simulink model "sm_flex_fe_import_beam_test"  (R2016a)
settings: Solver=ode23t  SolverMode=SingleTasking  StartTime=0.0  StopTime=tip_force_duration*2  RelTol=1e-3  AbsTol=1e-3
PreLoadFcn:
  | if(~exist('beamLink','var'))
  | sm_flex_fe_import_params
  | end
PostLoadFcn:
  | sm_flex_fe_import_beam_configure_load(bdroot,'Tip Load');
undefined symbols (not defined in the file): beamLink, gravity_vector, tip_force, tip_force_duration
libraries: nesl_utility x7, sm_lib x4, sm_flex_body_lib x1
CloseFcn:
  | try,close(h1_sm_flex_fe_import_beam),end
  | clear h1_sm_flex_fe_import_beam
  | try,close(h2_sm_flex_fe_import_beam),end
  | clear h2_sm_flex_fe_import_beam
  | try,close(h3_sm_flex_fe_import_beam),end
  | clear h3_sm_flex_fe_import_beam
  | try,close(h4_sm_flex_fe_import_beam),end
  | clear h4_sm_flex_fe_import_beam
  | 
  | 
  | clear simlog_sm_flex_fe_import_beam
  | clear logsout_sm_flex_fe_import_beam
Description:
  | Flexible Beam from Finite Element Data
  | 
  | Copyright 2016-2017 The MathWorks, Inc.
settings Model: Creator=yvanwedd  LastModifiedBy=smiller
settings DataIOCC: MaxDataPoints=25000  SignalLoggingName=logsout_sm_flex_fe_import_beam
settings DebuggingCC: SFUnexpectedBacktrackingDiag=error  SFNoUnconditionalDefaultTransitionDiag=error
settings GRTTargetCC: TargetLangStandard=C99 (ISO)  GeneratePreprocessorConditionals=Use local settings
settings ConfigComp: CovMetricSettings=dwe  CovHtmlReporting=off  CovSaveCumulativeToWorkspaceVar=off  CovSaveSingleToWorkspaceVar=off  CovExternalEMLEnable=on
settings SimscapeCC: SimscapeLogType=all  SimscapeLogSimulationStatistics=on  SimscapeLogName=simlog_sm_flex_fe_import_beam  SimscapeLogDataHistory=25000
settings ExplorerConfigSet: InternalSimMechanicsExplorerSettings="<ExplorerConfiguration><canonicalview>default</canonicalview><AnimationSetting><BasePlaybackSpeed>1.0</BasePlaybackSpeed><PlaybackSpeedFactor>4.0</PlaybackSpeedFactor></AnimationSetting><TilePanel><TileInfo><Tiles Columns=\"1\" Count=\"1\" Rows=\"1\"><Column Left=\"2\" Weight=\"1\"/><Column Left=\"597\"/><Row Top=\"2\" Weight=\"1\"/><Row Top=\"485\"/><Tile Height=\"1\" Width=\"1\" X=\"0\" Y=\"0\"/></Tiles></TileInfo><SceneInfo><SceneViewer><BGColor><R>1</R><G>1</G><B>1</B></BGColor><Camera><DoPerspective>off</DoPerspective><Position><X>1.1286167496242077</X><Y>0.14530787779879978</Y><Z>-0.1353875216555199</Z></Position><Center><X>0.14961601353852311</X><Y>-0.0070840019085978458</Y><Z>1.6591069809918091e-05</Z></Center><Up><X>-0.15237300927665429</X><Y>0.98826658924766431</Y><Z>0.010564782097399028</Z></Up><ViewLimDist>1</ViewLimDist><YLim>0.037474021129310135</YLim><XLim>0.046328642155645021</XLim></Camera></SceneViewer></SceneInfo></TilePanel><MechEditorPanel><Cameras/><GfxPanelCameraMap/><VideoCreator><PlaybackSpeedRatio>1.0</PlaybackSpeedRatio><FrameRate>30</FrameRate><VideoFormat>Motion JPEG AVI</VideoFormat><FrameSize>auto</FrameSize></VideoCreator></MechEditorPanel></ExplorerConfiguration>"

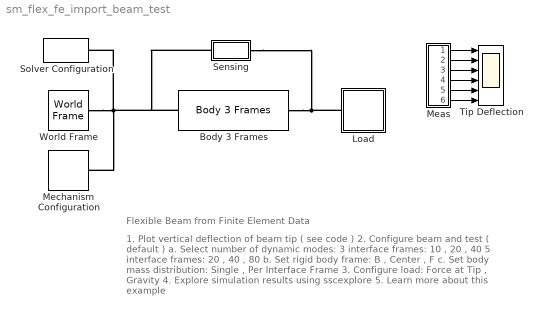
== system sm_flex_fe_import_beam_test ==
  note: Flexible Beam from Finite Element Data
  note: 1. Plot vertical deflection of beam tip ( see code )
      | 2. Configure beam and test ( default )
      | a. Select number of dynamic modes:
      | 3 interface frames: 10 , 20 , 40
      | 5 interface frames: 20 , 40 , 80
      | b. Set rigid body frame: B , Center , F
      | c. Set body mass distribution: Single , Per Interface Frame
      | 3. Configure load: Force at Tip , Gravity
      | 4. Explore simulation results using sscexplore
      | 5. Learn more about this example
  Body 3 Frames : sm_flex_body_lib/FE Import/Bodies/Body 3 Frames  popup_massdistr=Per Interface Frame  mass=beamLink.iner.mass  com=beamLink.iner.com  moi=beamLink.iner.moi  poi=beamLink.iner.poi  splitBodyProps=beamLink.splitBodyProps(2).props  smallInertiaDim=1e-3  smallInertiaMass=1e-6  rigid_body_filename='BeamLink.stl'  rigid_body_color=[0.0 0.4 0.6]  rigid_body_opacity=0  intf_body_color=[0.0 0.4 0.6]  intf_body_opacity=1  intf_graphic_color=[0.0 0.4 0.6]  intf_graphic_opacity=0  rigidBodyFrame=2  T=beamLink.models(5).T  numframes=3  K=beamLink.models(5).K  M=beamLink.models(5).M  ksi=0.05  dofIdxMap=beamLink.models(5).dofIdxMap  tau=1e-6  H=beamLink.models(5).H  sensedFeaDofs_UI=[]  numDynModes=20
      settings: AttributesFormatString=|
      | Mass: %<popup_massdistr>
      | Interface Frames: %<numframes>
      | Rigid Frame: %<rigidBodyFrame>
      | # Dynamic Modes: %<numDynModes>
  Load : Subsystem  mask{t1=0, t2=tip_force_duration, A=tip_force, loadDir=fy, coefs_dl=beamLink.coefs.cdf, coefs=beamLink.coefs.ctl, beam_mass=beamLink.iner.mass, grav_vector=gravity_vector}
      mask prompts: t1 "Start Time (sec)"; t2 "End Time (sec)"; A "Magnitude"; loadDir "Load Direction"; coefs_dl "Distributed Load Coefficients"; coefs "Tip Load Coefficients"; beam_mass "Beam Mass (kg)"; grav_vector "Gravity [x y z] (m/s^2)"
      mask init:
      | blk = [gcb '/External Force and Torque'];
      | mult_x = 0; mult_tx = 0;
      | mult_y = 0; mult_ty = 0;
      | mult_z = 0; mult_tz = 0;
      | 
      | switch loadDir
      |     case 1,
      |         set_param(blk, 'EnableForceX', 'on');
      |         set_param(blk, 'EnableForceY', 'off');
      |         set_param(blk, 'EnableForceZ', 'off');
      |         set_param(blk, 'EnableTorqueX', 'off');
      |         set_param(blk, 'EnableTorqueY', 'off');
      |         set_param(blk, 'EnableTorqueZ', 'off');
      |         mult_x = 1;
      |     case 2,
      |         set_param(blk, 'EnableForceY', 'on');
      |         set_param(blk, 'EnableForceX', 'off');
      |         set_param(blk, 'EnableForceZ', 'off');
      |         set_param(blk, 'EnableTorqueX', 'off');
      |         set_param(blk, 'EnableTorqueY', 'off');
      |         set_param(blk, 'EnableTorqueZ', 'off');
      |         mult_y = 1;
      |     case 3,
      |         set_param(blk, 'EnableForceZ', 'on');
      |         set_param(blk, 'EnableForceX', 'off');
      |         set_param(blk, 'EnableForceY', 'off');
      |         set_param(blk, 'EnableTorqueX', 'off');
      |         set_param(blk, 'EnableTorqueY', 'off');
      |         set_param(blk, 'EnableTorqueZ', 'off');
      |         mult_z = 1;
      |     case 4,
      |         set_param(blk, 'EnableTorqueX', 'on');
      |         set_param(blk, 'EnableForceX', 'off');
      |         set_param(blk, 'EnableForceY', 'off');
      |         set_param(blk, 'EnableForceZ', 'off');
      |         set_param(blk, 'EnableTorqueY', 'off');
      |         set_param(blk, 'EnableTorqueZ', 'off');
      |         mult_tx = 1;
      |     case 5,
      |         set_param(blk, 'EnableTorqueY', 'on');
      |         set_param(blk, 'EnableForceX', 'off');
      |         set_param(blk, 'EnableForceY', 'off');
      |         set_param(blk, 'EnableForceZ', 'off');
      |         set_param(blk, 'EnableTorqueX', 'off');
      |         set_param(blk, 'EnableTorqueZ', 'off');
      |         mult_ty = 1;
      |     case 6,
      |         set_param(blk, 'EnableTorqueZ', 'on');
      |         set_param(blk, 'EnableForceX', 'off');
      |         set_param(blk, 'EnableForceY', 'off');
      |         set_param(blk, 'EnableForceZ', 'off');
      |         set_param(blk, 'EnableTorqueX', 'off');
      |         set_param(blk, 'EnableTorqueY', 'off');
      |         mult_tz = 1;
      |     otherwise, assert(false);
      | end
      | 
      | blk = [gcb '/S-PS'];
      | 
      | if any(loadDir == [1 2 3])
      |     set_param(blk, 'Unit', 'N');
      | else
      |     set_param(blk, 'Unit', 'N*m');
      | end
      settings: AttributesFormatString=|
      | Amplitude: %<A>
      | Direction: %<loadDir>
      mask TypeOptions loadDir: fx | fy | fz | tx | ty | tz
  Meas : Subsystem
  Mechanism Configuration : sm_lib/Utilities/Mechanism Configuration  UniformGravity=None  GravityVector=gravity_vector  GravityUnits=m/s^2  LinearizationDelta=0.001
      settings: AttributesFormatString=Gravity: %<UniformGravity>
  Sensing : Subsystem
  Solver Configuration : nesl_utility/Solver Configuration  PhysicalDomain=network_engine_domain  SubClassName=solver  LeftPortType=input  RightPortType=generic  Accelerate=off  Tones=[]  Harmonics=[]  SimulateNoise=off  Profile=off  UseLocalSampling=off  EnableSwitchedLinearOptims=on  FrequencyDomain=off  UseCCode=off  RelTol=0.001  AbsTol=1e-06  MinStep=1e-09  ToWorkspace=off  RevertToSquareIcSolve=off  NumHomotopyIterations=100  PhasorMode=off  PhasorModeNumHarmonics=1  OverrideAbsTol=off  DoDC=off  ResidualTolerance=1e-09  UseLocalSolver=off  LocalSolverChoice=NE_BACKWARD_EULER_ADVANCER  LocalSolverSampleTime=0.001  DoFixedCost=off  MaxNonlinIter=3  MaxModeIter=2  LinearAlgebra=Sparse  DelaysMemoryBudget=1024  AutomaticFiltering=on  FilteringTimeConstant=0.001
  Tip Deflection : Scope  NumInputPorts=6
  World Frame : sm_lib/Frames and Transforms/World Frame
  wires:
  Meas/1(x) -> Tip Deflection/1
  Meas/2(y) -> Tip Deflection/2
  Meas/3(z) -> Tip Deflection/3
  Meas/4(qx) -> Tip Deflection/4
  Meas/5(qy) -> Tip Deflection/5
  Meas/6(qz) -> Tip Deflection/6
  connections:
  Body 3 Frames/LConn1 -- Sensing/LConn1 -- Mechanism Configuration/RConn1 -- Solver Configuration/RConn1 -- World Frame/RConn1
  Sensing/RConn1 -- Body 3 Frames/RConn1 -- Load/RConn1

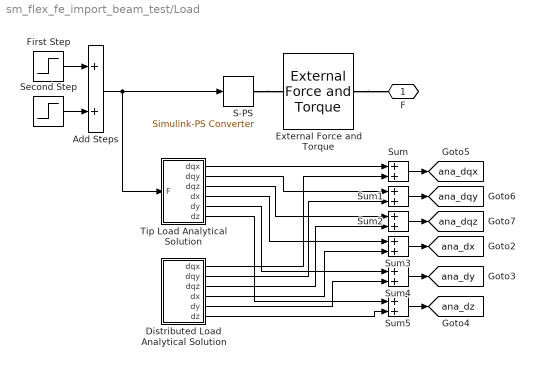
== system sm_flex_fe_import_beam_test/Load ==
  Add Steps : Sum
  Distributed Load Analytical Solution : Subsystem
  External Force and Torque : sm_lib/Forces and Torques/External Force and Torque  ForceResolutionFrame=World  EnableForceX=off  EnableForceY=on  EnableForceZ=off  EnableForce=off  TorqueResolutionFrame=World  EnableTorqueX=off  EnableTorqueY=off  EnableTorqueZ=off  EnableTorque=off
  First Step : Step  Time=t1  Before=-A  After=0  SampleTime=0
  S-PS : nesl_utility/Simulink-PS Converter  PhysicalDomain=network_engine_domain  SubClassName=ps_input  LeftPortType=input  RightPortType=output  PseudoPeriodic=off  Frequencies=[]  NoiseDistribution=none  NoiseParameters=[]  Unit=N  AffineConversion=off  InputFiltering=off  SimscapeFilterOrder=1  InputFilterTimeConstant=0.001  UdotUserProvided=1
  Second Step : Step  Time=t2  Before=A  After=0  SampleTime=0
  Sum{,1..5} (6 alike) : Sum
  Tip Load Analytical Solution : Subsystem
  F : PMIOPort  Port=1  Side=Right
  tag scope: ana_dqx=global, ana_dqy=global, ana_dqz=global, ana_dx=global, ana_dy=global, ana_dz=global
  wires:
  Add Steps/1 -> S-PS/1, Tip Load Analytical Solution/1(F)
  First Step/1 -> Add Steps/1
  Second Step/1 -> Add Steps/2
  Sum/1 -> [ana_dqx]
  Tip Load Analytical Solution/1(dqx) -> Sum/1
  Distributed Load Analytical Solution/1(dqx) -> Sum/2
  Sum1/1 -> [ana_dqy]
  Tip Load Analytical Solution/2(dqy) -> Sum1/1
  Distributed Load Analytical Solution/2(dqy) -> Sum1/2
  Sum2/1 -> [ana_dqz]
  Sum3/1 -> [ana_dx]
  Sum4/1 -> [ana_dy]
  Sum5/1 -> [ana_dz]
  Tip Load Analytical Solution/3(dqz) -> Sum2/1
  Distributed Load Analytical Solution/3(dqz) -> Sum2/2
  Tip Load Analytical Solution/4(dx) -> Sum3/1
  Distributed Load Analytical Solution/4(dx) -> Sum3/2
  Tip Load Analytical Solution/5(dy) -> Sum4/1
  Distributed Load Analytical Solution/5(dy) -> Sum4/2
  Tip Load Analytical Solution/6(dz) -> Sum5/1
  Distributed Load Analytical Solution/6(dz) -> Sum5/2
  connections:
  S-PS/RConn1 -- External Force and Torque/LConn1
  External Force and Torque/RConn1 -- F/RConn1

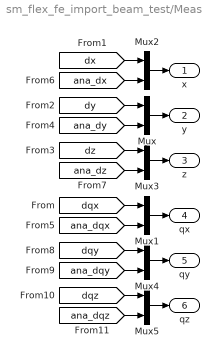
== system sm_flex_fe_import_beam_test/Meas ==
  Mux{,1..5} (6 alike) : Mux  Inputs=2
  x : Outport
  y : Outport  Port=2
  z : Outport  Port=3
  qx : Outport  Port=4
  qy : Outport  Port=5
  qz : Outport  Port=6
  wires:
  [ana_dz] -> Mux3/2
  [ana_dqy] -> Mux4/2
  [dqy] -> Mux4/1
  Mux4/1 -> qy/1
  [dqz] -> Mux5/1
  Mux/1 -> y/1
  Mux2/1 -> x/1
  Mux3/1 -> z/1
  [ana_dx] -> Mux2/2
  [dy] -> Mux/1
  [ana_dy] -> Mux/2
  Mux1/1 -> qx/1
  [dqx] -> Mux1/1
  [dx] -> Mux2/1
  [ana_dqx] -> Mux1/2
  [ana_dqz] -> Mux5/2
  Mux5/1 -> qz/1
  [dz] -> Mux3/1

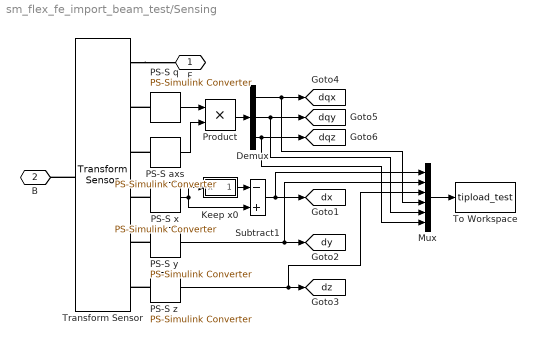
== system sm_flex_fe_import_beam_test/Sensing ==
  Demux : Demux  Outputs=3
  Keep x0 : Subsystem
  Mux : Mux  Inputs=6
  PS-S axs : nesl_utility/PS-Simulink Converter  PhysicalDomain=network_engine_domain  SubClassName=ps_output  LeftPortType=input  RightPortType=output  PseudoPeriodic=off  Frequencies=[]  Unit=1  AffineConversion=off
  PS-S q : nesl_utility/PS-Simulink Converter  PhysicalDomain=network_engine_domain  SubClassName=ps_output  LeftPortType=input  RightPortType=output  PseudoPeriodic=off  Frequencies=[]  Unit=rad  AffineConversion=off
  PS-S x : nesl_utility/PS-Simulink Converter  PhysicalDomain=network_engine_domain  SubClassName=ps_output  LeftPortType=input  RightPortType=output  PseudoPeriodic=off  Frequencies=[]  Unit=m  AffineConversion=off
  PS-S y : nesl_utility/PS-Simulink Converter  PhysicalDomain=network_engine_domain  SubClassName=ps_output  LeftPortType=input  RightPortType=output  PseudoPeriodic=off  Frequencies=[]  Unit=m  AffineConversion=off
  PS-S z : nesl_utility/PS-Simulink Converter  PhysicalDomain=network_engine_domain  SubClassName=ps_output  LeftPortType=input  RightPortType=output  PseudoPeriodic=off  Frequencies=[]  Unit=m  AffineConversion=off
  Product : Product
  Subtract1 : Sum  Inputs=-+
  To Workspace : ToWorkspace  VariableName=tipload_test  SaveFormat=Timeseries  SampleTime=-1
  Transform Sensor : sm_lib/Frames and Transforms/Transform Sensor  MeasurementFrame=World  SenseAngle=on  SenseAxis=on  SenseAngle1=off  SenseAngle2=off  SenseAngle3=off  SenseQ=off  SenseR=off  SenseOmegaX=off  SenseOmegaY=off  SenseOmegaZ=off  SenseOmega1=off  SenseOmega2=off  SenseOmega3=off  SenseQDot=off  SenseRDot=off  SenseAlphaX=off  SenseAlphaY=off  SenseAlphaZ=off  SenseAlpha1=off  SenseAlpha2=off  SenseAlpha3=off  SenseQDDot=off  SenseRDDot=off  SenseX=on  SenseY=on  SenseZ=on  SenseRad=off  SenseAzim=off  SenseDist=off  SenseInc=off  SenseXDot=off  SenseYDot=off  SenseZDot=off  SenseRadDot=off  SenseAzimDot=off  SenseDistDot=off  SenseIncDot=off  SenseXDDot=off  SenseYDDot=off  SenseZDDot=off  SenseRadDDot=off  SenseAzimDDot=off  SenseDistDDot=off  SenseIncDDot=off
  F : PMIOPort  Port=1  Side=Right
  B : PMIOPort  Port=2  Side=Left
  tag scope: dqx=global, dqy=global, dqz=global, dx=global, dy=global, dz=global
  wires:
  PS-S axs/1 -> Product/2
  PS-S q/1 -> Product/1
  PS-S z/1 -> [dz], Mux/3
  PS-S y/1 -> [dy], Mux/2
  Mux/1 -> To Workspace/1
  Product/1 -> Demux/1
  Demux/1 -> Mux/4, [dqx]
  Demux/2 -> [dqy], Mux/5
  Demux/3 -> Mux/6, [dqz]
  Subtract1/1 -> [dx], Mux/1
  PS-S x/1 -> Keep x0/1(x), Subtract1/2
  Keep x0/1(x0) -> Subtract1/1
  connections:
  PS-S y/LConn1 -- Transform Sensor/RConn5
  PS-S axs/LConn1 -- Transform Sensor/RConn3
  Transform Sensor/RConn1 -- F/RConn1
  PS-S q/LConn1 -- Transform Sensor/RConn2
  Transform Sensor/LConn1 -- B/RConn1
  PS-S x/LConn1 -- Transform Sensor/RConn4
  PS-S z/LConn1 -- Transform Sensor/RConn6

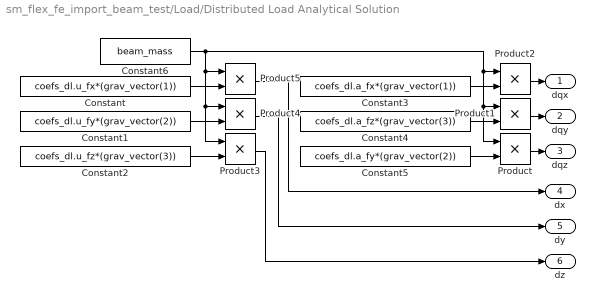
== system sm_flex_fe_import_beam_test/Load/Distributed Load Analytical Solution ==
  Constant : Constant  Value=coefs_dl.u_fx*(grav_vector(1))
  Constant1 : Constant  Value=coefs_dl.u_fy*(grav_vector(2))
  Constant2 : Constant  Value=coefs_dl.u_fz*(grav_vector(3))
  Constant3 : Constant  Value=coefs_dl.a_fx*(grav_vector(1))
  Constant4 : Constant  Value=coefs_dl.a_fz*(grav_vector(3))
  Constant5 : Constant  Value=coefs_dl.a_fy*(grav_vector(2))
  Constant6 : Constant  Value=beam_mass
  Product{,1..5} (6 alike) : Product
  dqx : Outport
  dqy : Outport  Port=2
  dqz : Outport  Port=3
  dx : Outport  Port=4
  dy : Outport  Port=5
  dz : Outport  Port=6
  wires:
  Constant1/1 -> Product4/2
  Product5/1 -> dx/1
  Product3/1 -> dz/1
  Product1/1 -> dqy/1
  Product4/1 -> dy/1
  Product/1 -> dqz/1
  Constant4/1 -> Product1/2
  Constant5/1 -> Product/2
  Constant2/1 -> Product3/2
  Constant3/1 -> Product2/2
  Product2/1 -> dqx/1
  Constant/1 -> Product5/2
  Constant6/1 -> Product5/1, Product4/1, Product3/1, Product/1, Product1/1, Product2/1

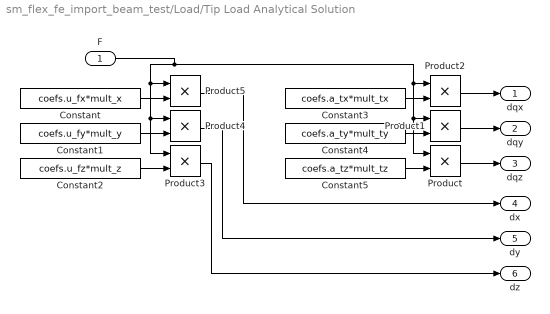
== system sm_flex_fe_import_beam_test/Load/Tip Load Analytical Solution ==
  F : Inport
  Constant : Constant  Value=coefs.u_fx*mult_x
  Constant1 : Constant  Value=coefs.u_fy*mult_y
  Constant2 : Constant  Value=coefs.u_fz*mult_z
  Constant3 : Constant  Value=coefs.a_tx*mult_tx
  Constant4 : Constant  Value=coefs.a_ty*mult_ty
  Constant5 : Constant  Value=coefs.a_tz*mult_tz
  Product{,1..5} (6 alike) : Product
  dqx : Outport
  dqy : Outport  Port=2
  dqz : Outport  Port=3
  dx : Outport  Port=4
  dy : Outport  Port=5
  dz : Outport  Port=6
  wires:
  F/1 -> Product3/1, Product4/1, Product5/1, Product2/1, Product1/1, Product/1
  Constant/1 -> Product5/2
  Product2/1 -> dqx/1
  Constant3/1 -> Product2/2
  Constant2/1 -> Product3/2
  Constant5/1 -> Product/2
  Constant4/1 -> Product1/2
  Product/1 -> dqz/1
  Product4/1 -> dy/1
  Product1/1 -> dqy/1
  Product3/1 -> dz/1
  Product5/1 -> dx/1
  Constant1/1 -> Product4/2

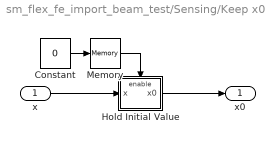
== system sm_flex_fe_import_beam_test/Sensing/Keep x0 ==
  x : Inport
  Constant : Constant  Value=0
  Hold Initial Value : Subsystem
  Memory : Memory  X0=1
  x0 : Outport
  wires:
  Constant/1 -> Memory/1
  Hold Initial Value/1(x0) -> x0/1
  x/1 -> Hold Initial Value/1(x)
  Memory/1 -> Hold Initial Value/Enable

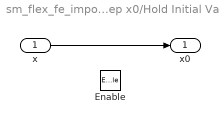
== system sm_flex_fe_import_beam_test/Sensing/Keep x0/Hold Initial Value ==
  x : Inport
  Enable : EnablePort
  x0 : Outport
  wires:
  x/1 -> x0/1
